simulink model "observer_controller_model_arduino"  (R2020a)
settings: Solver=VariableStepAuto  StartTime=0.0  StopTime=ref(end,1)  RelTol=1e-3
values from neighbouring files (symbols this model uses):
  C = Ad.C    [Observer_mat.m]    (also in discretemodel.mat = [0  0  1  0; 0  0  0  1]; lqr_whitebox.m = sys.C; lqr_whitebox.mat = [0  0  1  0; 0  0  0  1]; matrices.mat = [0  0  1  0; 0  0  0  1])
  gamma = Ad.B    [Observer_mat.m]    (also in discretemodel.mat = [0.004353030085  4.48398112985e-06; 6.47055504813e-06  0.003; observer_matlab.m; observermatlab.m)
  h = tout(2)-tout(1)    [Linearize_whitebox.m]    (also in Linearize_whitebox_final.m; Observer_mat.m; lqr_whitebox.mat = 1.00037043897; matrices.mat = 1.00080032013)
  K = [0.871464143609  0.0262786205748; 0.0262786205748  0.871464143609; 0.341518856741  0.00295216925623; 0.00295216925623  0.341518856741]    [K_matrix.mat]    (also in K_matrix_final.mat = [0.107540648809  0.00297468629139; 0.00297468629139  0.10754; Observer_mat.m = place(phi.',C.',P).'; lqr_whitebox.m = lqr(A,B,Q,R); lqr_whitebox.mat = [9.8403850338  0.823629600444  7.09136571585  0.104667034235)
  L = lqr(A,B,Q,R)    [LQR.m]    (also in LQR_final.m; L_Lr_LQR.mat = [210.936834033  1.0429491506  82.9532479278  0.141237062686;; L_Lr_LQR_final.mat = [15.3959700225  0.0810970521206  45.9635678787  0.9358925165; L_Lr_Pole_Placement.mat = [382.498734136  0.681043508792  3740.11964319  0; 0.98277164)
  Lr = inv(Ldc)    [LQR.m]    (also in LQR_final.m; L_Lr_LQR.mat = [295.811652311  0.50314270449; -0.353029029898  433.02182351; L_Lr_LQR_final.mat = [63.2811082521  0.33594605992; -0.399513584683  63.309082518; L_Lr_Pole_Placement.mat = [4124.53994767  0; 0  5951.86777259])
  phi = Ad.A    [Observer_mat.m]    (also in discretemodel.mat = [0.991639753181 0.00295216925623 0.0399517774449 5.979211225; observer_matlab.m; observermatlab.m)
undefined symbols (not defined in the file or in its folder): init_temp
libraries: simulink x1
settings Model: Creator=SIDTUDelft1  LastModifiedBy=SIDTUDelft1

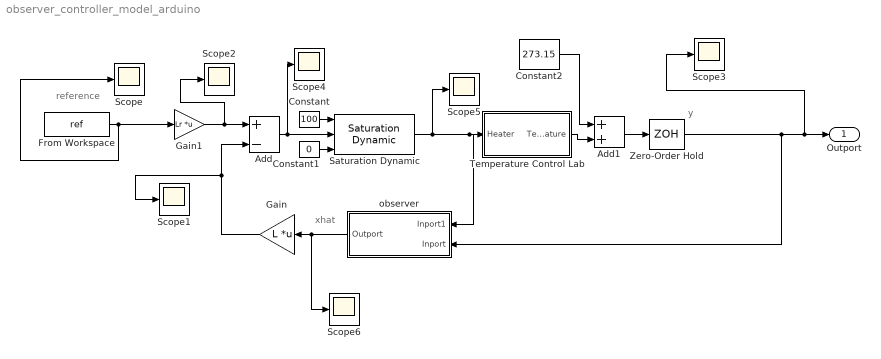
== system observer_controller_model_arduino ==
  note: reference
  note: y
  note: xhat
  Add : Sum  Inputs=+-  OutMin=[0]  OutMax=[100]
  Add1 : Sum
  Constant : Constant  Value=100
  Constant1 : Constant  Value=0
  Constant2 : Constant  Value=273.15
  From Workspace : FromWorkspace  VariableName=ref  SampleTime=h
  Gain : Gain  Gain=L  Multiplication=Matrix(K*u)
  Gain1 : Gain  Gain=Lr  Multiplication=Matrix(K*u)
  Saturation Dynamic : simulink/Discontinuities/Saturation Dynamic  OutMin=[0]  OutMax=[100]  OutDataTypeStr=Inherit: Same as second input  OutDataType=fixdt(1, 16)  OutScaling=2^-10  DoSatur=off
  Scope{,1..6} (7 alike) : Scope
  Temperature Control Lab : Subsystem
  Zero-Order Hold : ZeroOrderHold  SampleTime=h
  observer : Subsystem
  Outport : Outport
  wires:
  observer/1(Outport) -> Scope6/1, Gain/1
  Gain1/1 -> Scope2/1, Add/1
  From Workspace/1 -> Scope/1, Gain1/1
  Add/1 -> Scope4/1, Saturation Dynamic/2
  Saturation Dynamic/1 -> Scope5/1, observer/1(Inport1), Temperature Control Lab/1(Heater)
  Constant/1 -> Saturation Dynamic/1
  Constant1/1 -> Saturation Dynamic/3
  Temperature Control Lab/1(Temperature) -> Add1/2
  Constant2/1 -> Add1/1
  Gain/1 -> Scope1/1, Add/2
  Add1/1 -> Zero-Order Hold/1
  Zero-Order Hold/1 -> observer/2(Inport), Scope3/1, Outport/1

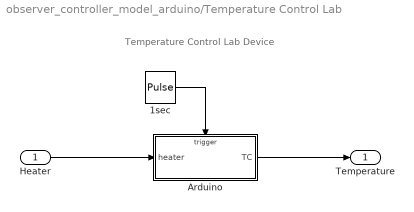
== system observer_controller_model_arduino/Temperature Control Lab ==
  note: Temperature Control Lab Device
  Heater : Inport
  1sec : DiscretePulseGenerator  PulseType=Time based  Period=1  PulseWidth=50
  Arduino : Subsystem  TreatAsAtomicUnit=on
  Temperature : Outport
  wires:
  1sec/1 -> Arduino/Trigger
  Arduino/1(TC) -> Temperature/1
  Heater/1 -> Arduino/1(heater)

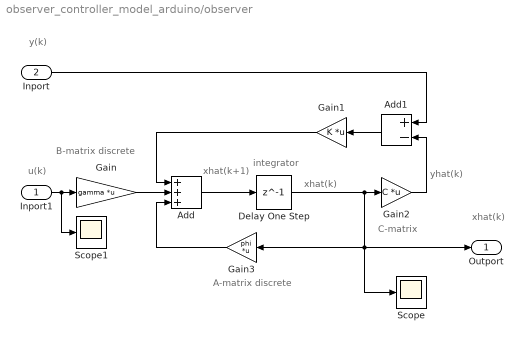
== system observer_controller_model_arduino/observer ==
  note: C-matrix
  note: B-matrix discrete
  note: A-matrix discrete
  note: yhat(k)
  note: xhat(k+1)
  note: y(k)
  note: xhat(k)
  note: u(k)
  note: xhat(k)
  note: integrator
  Inport1 : Inport
  Inport : Inport  Port=2
  Add : Sum  Inputs=+++
  Add1 : Sum  Inputs=+-
  Delay One Step : Delay  DelayLength=1  InitialCondition=init_temp  SampleTime=h
  Gain : Gain  Gain=gamma  Multiplication=Matrix(K*u)
  Gain1 : Gain  Gain=K  Multiplication=Matrix(K*u)
  Gain2 : Gain  Gain=C  Multiplication=Matrix(K*u)
  Gain3 : Gain  Gain=phi  Multiplication=Matrix(K*u)
  Scope : Scope
  Scope1 : Scope
  Outport : Outport
  wires:
  Add/1 -> Delay One Step/1
  Add1/1 -> Gain1/1
  Gain1/1 -> Add/1
  Gain/1 -> Add/2
  Gain2/1 -> Add1/2
  Gain3/1 -> Add/3
  Inport/1 -> Add1/1
  Inport1/1 -> Scope1/1, Gain/1
  Delay One Step/1 -> Gain3/1, Scope/1, Outport/1, Gain2/1

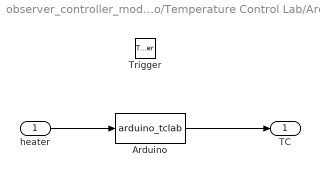
== system observer_controller_model_arduino/Temperature Control Lab/Arduino ==
  heater : Inport  LatchByDelayingOutsideSignal=on
  Trigger : TriggerPort  VariantControl=Variant
  Arduino : MATLABFcn  MATLABFcn=arduino_tclab
  TC : Outport  InitialOutput=23
  wires:
  heater/1 -> Arduino/1
  Arduino/1 -> TC/1
